simulink model "testbench_with_kalmanfilter"  (R2016a)
settings: Solver=FixedStepAuto  StartTime=0.0  StopTime=10  RelTol=1e-3
values from neighbouring files (symbols this model uses):
  A = [1 1 0;0 1 1;0 0 1]    [kalman_script.m]
undefined symbols (not defined in the file or in its folder): Discrete, Time
libraries: legoev3lib x4, ctrlSharedLib x1
settings Model: SimulationMode=external  ExtModeTrigDuration=2  Creator=Shobhit  LastModifiedBy=Shobhit
settings SolverCC: PositivePriorityOrder=on
settings OptimizationCC: OptimizeModelRefInitCode=on  LifeSpan=1  MaxStackSize=64
settings HardwareCC: ProdBitPerPointer=32  ProdLargestAtomicInteger=Long  ProdWordSize=32  ProdHWDeviceType=ARM Compatible->ARM 9  UseEmbeddedCoderFeatures=off  UseSimulinkCoderFeatures=off
settings RTWCC: SystemTargetFile=ert.tlc  HardwareBoard=LEGO MINDSTORMS EV3  TemplateMakefile=ert_default_tmf  GenerateReport=on  Toolchain=Sourcery G++ Lite v2009q3  IncludeHyperlinkInReport=on  LaunchReport=on  GenerateTraceInfo=on  GenerateTraceReport=on  GenerateTraceReportSl=on  GenerateTraceReportSf=on  GenerateTraceReportEml=on
settings CodeAppCC: ForceParamTrailComments=on  IgnoreCustomStorageClasses=off  OperatorAnnotations=on  SimulinkDataObjDesc=on  SFDataObjDesc=on  MATLABFcnDesc=on  InsertBlockDesc=on  MATLABSourceComments=on
settings ERTTargetCC: SupportContinuousTime=on  SupportNonInlinedSFcns=on  SupportVariableSizeSignals=on

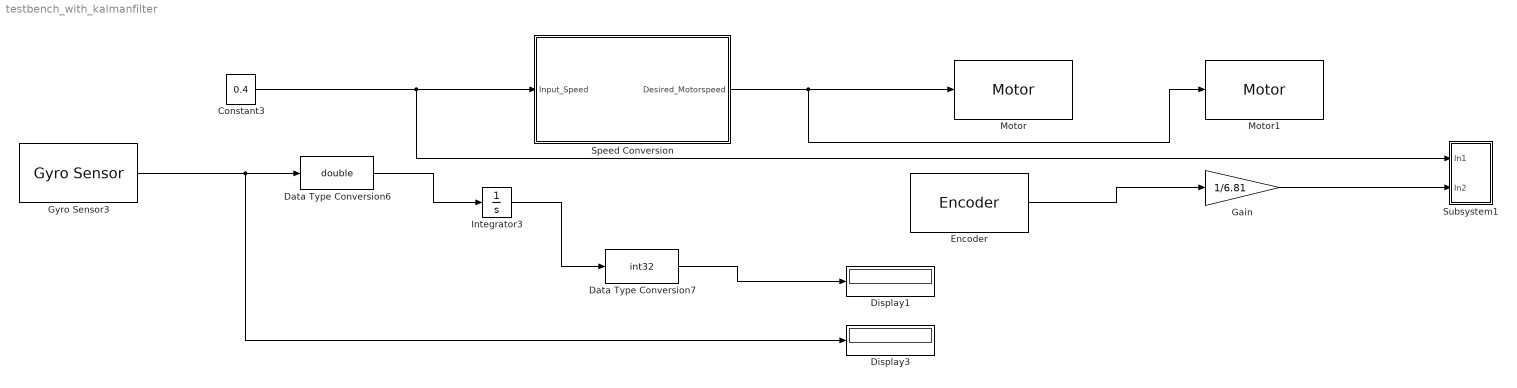
== system testbench_with_kalmanfilter ==
  Constant3 : Constant  Value=0.4
  Data Type Conversion6 : DataTypeConversion  OutDataTypeStr=double  RndMeth=Ceiling
  Data Type Conversion7 : DataTypeConversion  OutDataTypeStr=int32  RndMeth=Ceiling
  Display1 : Display
  Display3 : Display
  Encoder : legoev3lib/Encoder  portNumber=B  opMode=No reset  sampleTime=0.1
  Gain : Gain  Gain=1/6.81
  Gyro Sensor3 : legoev3lib/Gyro Sensor  portNumber=2  sampleTime=0.1
  Integrator3 : Integrator
  Motor : legoev3lib/Motor  sportNumber=A  sstopAction=Brake
  Motor1 : legoev3lib/Motor  sportNumber=B  sstopAction=Brake
  Speed Conversion : Subsystem
  Subsystem1 : Subsystem
  wires:
  Integrator3/1 -> Data Type Conversion7/1
  Data Type Conversion6/1 -> Integrator3/1
  Gyro Sensor3/1 -> Display3/1, Data Type Conversion6/1
  Speed Conversion/1(Desired_Motorspeed) -> Motor1/1, Motor/1
  Constant3/1 -> Subsystem1/1(In1), Speed Conversion/1(Input_Speed)
  Data Type Conversion7/1 -> Display1/1
  Encoder/1 -> Gain/1
  Gain/1 -> Subsystem1/2(In2)

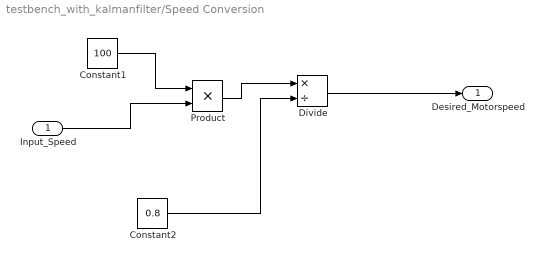
== system testbench_with_kalmanfilter/Speed Conversion ==
  Input_Speed : Inport
  Constant1 : Constant  Value=100
  Constant2 : Constant  Value=0.8
  Divide : Product  Inputs=*/
  Product : Product
  Desired_Motorspeed : Outport
  wires:
  Divide/1 -> Desired_Motorspeed/1
  Input_Speed/1 -> Product/2
  Constant2/1 -> Divide/2
  Product/1 -> Divide/1
  Constant1/1 -> Product/1

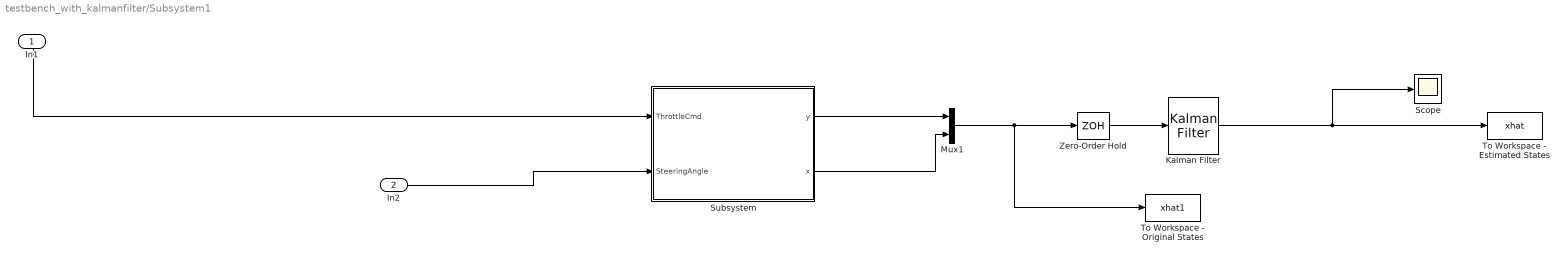
== system testbench_with_kalmanfilter/Subsystem1 ==
  In1 : Inport
  In2 : Inport  Port=2
  Kalman Filter : ctrlSharedLib/Kalman Filter  TimeDomain=Discrete-Time  UseCurrentEstimator=on  ModelSource=Individual A, B, C, D matrices  ModelSourceVariable=sys  A=A  B=1  C=[1 0 0;0 0 1]  D=0  NumberOfStates=1  NumberOfInputs=1  NumberOfOutputs=1  InitialEstimateSource=Dialog  X0=0  P0=10  UseK=off  UseGH=on  NumberOfProcessNoiseInputs=1  G=[1 0 0; 0 1 0;0 0 1]  TimeInvariantG=on  H=0  TimeInvariantH=on  Q=0.01  TimeInvariantQ=on  R=10  TimeInvariantR=on  N=0  TimeInvariantN=on  AddInputPort=off  AddEnablePort=off  OutputEstimatedY=off  OutputP=off  Ts=-1
  Mux1 : Mux  Inputs=2
  Scope : Scope
  Subsystem : Subsystem
  To Workspace - Estimated States : ToWorkspace  VariableName=xhat  SampleTime=-1
      settings: Save2DSignal=2-D array (concatenate along first dimension)
  "To Workspace - Original States " : ToWorkspace  VariableName=xhat1  SampleTime=-1
      settings: Save2DSignal=2-D array (concatenate along first dimension)
  Zero-Order Hold : ZeroOrderHold
  wires:
  Subsystem/2(x) -> Mux1/2
  Subsystem/1(y) -> Mux1/1
  Mux1/1 -> "To Workspace - Original States "/1, Zero-Order Hold/1
  Kalman Filter/1 -> Scope/1, To Workspace - Estimated States/1
  Zero-Order Hold/1 -> Kalman Filter/1
  In2/1 -> Subsystem/2(SteeringAngle)
  In1/1 -> Subsystem/1(ThrottleCmd)

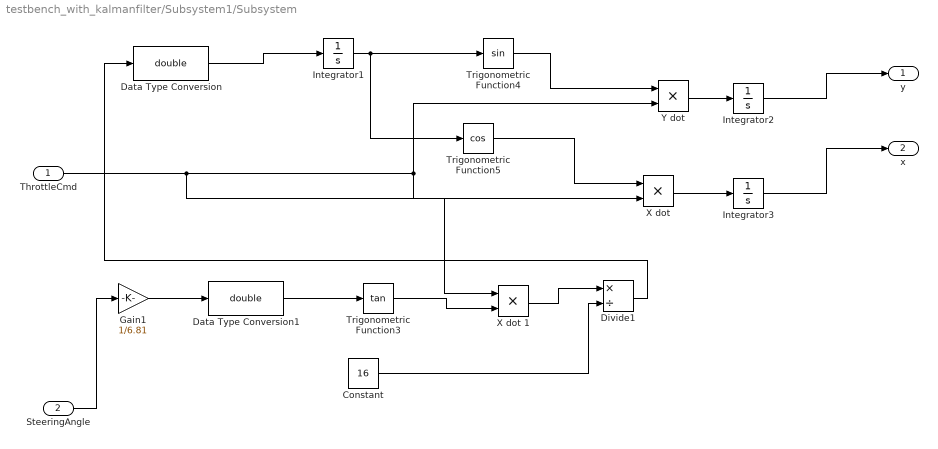
== system testbench_with_kalmanfilter/Subsystem1/Subsystem ==
  ThrottleCmd : Inport
  SteeringAngle : Inport  Port=2
  Constant : Constant  Value=16
  Data Type Conversion : DataTypeConversion  OutDataTypeStr=double
  Data Type Conversion1 : DataTypeConversion  OutDataTypeStr=double
  Divide1 : Product  Inputs=*/
  Gain1 : Gain  Gain=1/6.81
  Integrator1 : Integrator
  Integrator2 : Integrator
  Integrator3 : Integrator
  Trigonometric Function3 : Trigonometry  Operator=tan  OutputSignalType=real
  Trigonometric Function4 : Trigonometry
  Trigonometric Function5 : Trigonometry  Operator=cos
  "X dot " : Product
  X dot 1 : Product
  "Y dot " : Product
  y : Outport
  x : Outport  Port=2
  wires:
  Gain1/1 -> Data Type Conversion1/1
  Integrator1/1 -> Trigonometric Function5/1, Trigonometric Function4/1
  ThrottleCmd/1 -> X dot 1/1, "X dot "/2, "Y dot "/2
  Trigonometric Function5/1 -> "X dot "/1
  Trigonometric Function4/1 -> "Y dot "/1
  "X dot "/1 -> Integrator3/1
  "Y dot "/1 -> Integrator2/1
  Data Type Conversion/1 -> Integrator1/1
  Integrator2/1 -> y/1
  Integrator3/1 -> x/1
  SteeringAngle/1 -> Gain1/1
  Data Type Conversion1/1 -> Trigonometric Function3/1
  Constant/1 -> Divide1/2
  Divide1/1 -> Data Type Conversion/1
  Trigonometric Function3/1 -> X dot 1/2
  X dot 1/1 -> Divide1/1
